simulink model "RL_TTS3_System_Blank"  (R2019b)
settings: Solver=FixedStepAuto  StartTime=0.0  StopTime=10.0  FixedStep=0.01  RelTol=1e-3
undefined symbols (not defined in the file or in its folder): tubeSpeed1, tubeSpeed2
settings Model: Creator=rdkluijv  LastModifiedBy=edtve
settings DebuggingCC: BusObjectLabelMismatch=none
settings SFSimCC: CustomCodeUndefinedFunction=UseInterfaceOnly
settings CodeAppCC: MaxIdLength=63

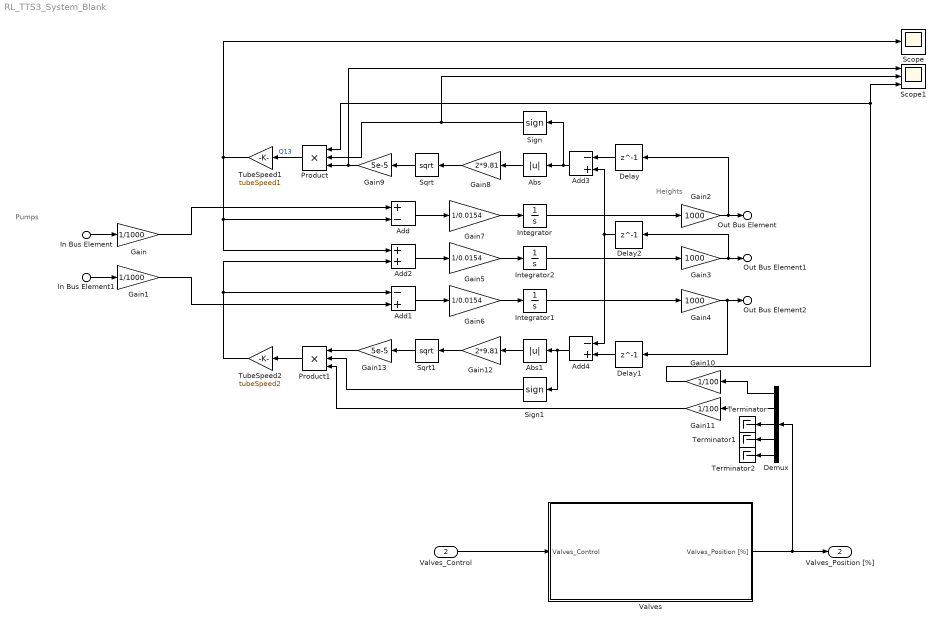
== system RL_TTS3_System_Blank ==
  note: Heights
  note: Pumps
  In Bus Element : Inport  PortName=Pumps [l/s]  Element=Left
  In Bus Element1 : Inport  PortName=Pumps [l/s]  Element=Right
  Valves_Control : Inport  Port=2  OutDataTypeStr=Bus: ValvesSICO
  Abs : Abs
  Abs1 : Abs
  Add : Sum  Inputs=+-
  Add1 : Sum  Inputs=-+
  Add2 : Sum
  Add3 : Sum  Inputs=-+
  Add4 : Sum  Inputs=-+
  Delay : Delay  DelayLength=1
  Delay1 : Delay  DelayLength=1
  Delay2 : Delay  DelayLength=1
  Demux : Demux  Outputs=5
  Gain : Gain  Gain=1/1000
  Gain1 : Gain  Gain=1/1000
  Gain10 : Gain  Gain=1/100
  Gain11 : Gain  Gain=1/100
  Gain12 : Gain  Gain=2*9.81
  Gain13 : Gain  Gain=5e-5
  Gain2 : Gain  Gain=1000
  Gain3 : Gain  Gain=1000
  Gain4 : Gain  Gain=1000
  Gain5 : Gain  Gain=1/0.0154
  Gain6 : Gain  Gain=1/0.0154
  Gain7 : Gain  Gain=1/0.0154
  Gain8 : Gain  Gain=2*9.81
  Gain9 : Gain  Gain=5e-5
  Integrator : Integrator
  Integrator1 : Integrator
  Integrator2 : Integrator
  Product : Product  Inputs=3
  Product1 : Product  Inputs=3
  Scope : Scope
  Scope1 : Scope  NumInputPorts=3
  Sign : Signum
  Sign1 : Signum
  Sqrt : Sqrt  SaturateOnIntegerOverflow=on
  Sqrt1 : Sqrt  SaturateOnIntegerOverflow=on
  Terminator : Terminator
  Terminator1 : Terminator
  Terminator2 : Terminator
  TubeSpeed1 : Gain  Gain=tubeSpeed1
  TubeSpeed2 : Gain  Gain=tubeSpeed2
  Valves : Subsystem  TreatAsAtomicUnit=on
  Out Bus Element : Outport  VectorParamsAs1DForOutWhenUnconnected=off  PortName=Heights [mm]  Element=Left
  Out Bus Element1 : Outport  VectorParamsAs1DForOutWhenUnconnected=off  PortName=Heights [mm]  Element=Middle
  Out Bus Element2 : Outport  VectorParamsAs1DForOutWhenUnconnected=off  PortName=Heights [mm]  Element=Right
  Valves_Position [%] : Outport  Port=2  OutDataTypeStr=Bus: ValvesSOCI
  wires:
  Valves_Control/1 -> Valves/1(Valves_Control)
  Valves/1(Valves_Position [%]) -> Demux/1, Valves_Position [%]/1
  In Bus Element/1 -> Gain/1
  In Bus Element1/1 -> Gain1/1
  Gain4/1 -> Delay1/1, Out Bus Element2/1
  Gain3/1 -> Delay2/1, Out Bus Element1/1
  Gain2/1 -> Delay/1, Out Bus Element/1
  Product1/1 -> TubeSpeed2/1
  Add2/1 -> Gain5/1
  Add1/1 -> Gain6/1
  Add/1 -> Gain7/1
  Gain7/1 -> Integrator/1
  Gain6/1 -> Integrator1/1
  Gain5/1 -> Integrator2/1
  Gain/1 -> Add/1
  Delay/1 -> Add3/1
  Add3/1 -> Sign/1, Abs/1
  Gain8/1 -> Sqrt/1
  Sqrt/1 -> Gain9/1
  Demux/3 -> Terminator/1
  Demux/4 -> Terminator1/1
  Demux/5 -> Terminator2/1
  Demux/1 -> Gain10/1
  Demux/2 -> Gain11/1
  Gain9/1 -> Product/3, Scope1/1
  Gain10/1 -> Scope1/3, Product/1
  Product/1 -> TubeSpeed1/1  "Q13"
  Add4/1 -> Sign1/1, Abs1/1
  Gain12/1 -> Sqrt1/1
  Sqrt1/1 -> Gain13/1
  Gain13/1 -> Product1/1
  Integrator/1 -> Gain2/1
  Abs/1 -> Gain8/1
  Abs1/1 -> Gain12/1
  Sign/1 -> Scope1/2, Product/2
  Sign1/1 -> Product1/2
  Integrator2/1 -> Gain3/1
  Integrator1/1 -> Gain4/1
  Delay2/1 -> Add4/1, Add3/2
  Delay1/1 -> Add4/2
  Gain11/1 -> Product1/3
  Gain1/1 -> Add1/2
  TubeSpeed2/1 -> Add2/2, Add1/1
  TubeSpeed1/1 -> Scope/1, Add/2, Add2/1

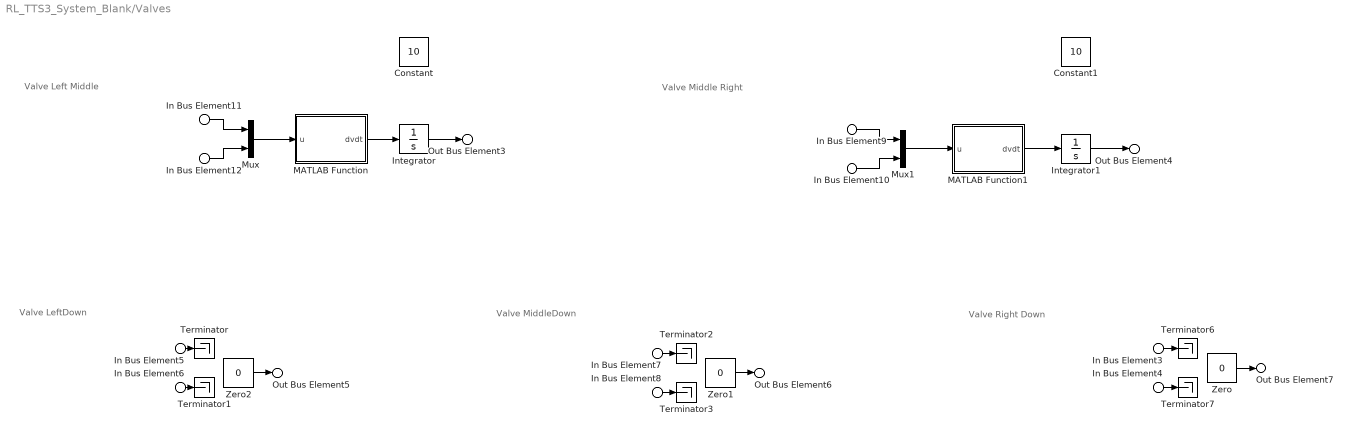
== system RL_TTS3_System_Blank/Valves ==
  note: Valve Right Down
  note: Valve Left Middle
  note: Valve Middle Right
  note: Valve MiddleDown
  note: Valve LeftDown
  In Bus Element3 : Inport  PortName=Valves_Control  Element=RightDown.Open
  In Bus Element4 : Inport  PortName=Valves_Control  Element=RightDown.Close
  In Bus Element5 : Inport  PortName=Valves_Control  Element=LeftDown.Open
  In Bus Element6 : Inport  PortName=Valves_Control  Element=LeftDown.Close
  In Bus Element7 : Inport  PortName=Valves_Control  Element=MiddleDown.Open
  In Bus Element8 : Inport  PortName=Valves_Control  Element=MiddleDown.Close
  In Bus Element9 : Inport  PortName=Valves_Control  Element=MiddleRight.Open
  In Bus Element10 : Inport  PortName=Valves_Control  Element=MiddleRight.Close
  In Bus Element11 : Inport  PortName=Valves_Control  Element=LeftMiddle.Open
  In Bus Element12 : Inport  PortName=Valves_Control  Element=LeftMiddle.Close
  Constant : Constant  Value=10
  Constant1 : Constant  Value=10
  Integrator : Integrator
  Integrator1 : Integrator
  MATLAB Function : MATLAB Function  TreatAsAtomicUnit=on
  MATLAB Function1 : MATLAB Function  TreatAsAtomicUnit=on
  Mux : Mux  Inputs=2
  Mux1 : Mux  Inputs=2
  Terminator{,1..3,6..7} (6 alike) : Terminator
  Zero : Constant  Value=0  OutDataTypeStr=Inherit: Inherit via back propagation
  Zero1 : Constant  Value=0  OutDataTypeStr=Inherit: Inherit via back propagation
  Zero2 : Constant  Value=0  OutDataTypeStr=Inherit: Inherit via back propagation
  Out Bus Element3 : Outport  VectorParamsAs1DForOutWhenUnconnected=off  PortName=Valves_Position [%]  Element=LeftMiddle
  Out Bus Element4 : Outport  VectorParamsAs1DForOutWhenUnconnected=off  PortName=Valves_Position [%]  Element=MiddleRight
  Out Bus Element5 : Outport  VectorParamsAs1DForOutWhenUnconnected=off  PortName=Valves_Position [%]  Element=LeftDown
  Out Bus Element6 : Outport  VectorParamsAs1DForOutWhenUnconnected=off  PortName=Valves_Position [%]  Element=MiddleDown
  Out Bus Element7 : Outport  VectorParamsAs1DForOutWhenUnconnected=off  PortName=Valves_Position [%]  Element=RightDown
  wires:
  Zero/1 -> Out Bus Element7/1
  Zero1/1 -> Out Bus Element6/1
  Zero2/1 -> Out Bus Element5/1
  In Bus Element5/1 -> Terminator/1
  In Bus Element6/1 -> Terminator1/1
  In Bus Element7/1 -> Terminator2/1
  In Bus Element8/1 -> Terminator3/1
  In Bus Element3/1 -> Terminator6/1
  In Bus Element4/1 -> Terminator7/1
  MATLAB Function/1(dvdt) -> Integrator/1
  MATLAB Function1/1(dvdt) -> Integrator1/1
  In Bus Element11/1 -> Mux/1
  Mux/1 -> MATLAB Function/1(u)
  In Bus Element12/1 -> Mux/2
  Mux1/1 -> MATLAB Function1/1(u)
  In Bus Element9/1 -> Mux1/1
  In Bus Element10/1 -> Mux1/2
  Integrator/1 -> Out Bus Element3/1
  Integrator1/1 -> Out Bus Element4/1

== matlab function RL_TTS3_System_Blank/Valves/MATLAB Function1 ==
  data: u input; dvdt output
function dvdt = fcn(u)

    if u(1)==false && u(2)==false
        dvdt = 0;
    elseif u(1)==false && u(2)==true
        dvdt = -100/9;
    elseif u(1)==true && u(2)==false
        dvdt = 100/9;
    else
        dvdt=0;
    end
    
end

== matlab function RL_TTS3_System_Blank/Valves/MATLAB Function ==
  data: u input; dvdt output
function dvdt = fcn(u)

    if u(1)==false && u(2)==false
        dvdt = 0;
    elseif u(1)==false && u(2)==true
        dvdt = -100/9;
    elseif u(1)==true && u(2)==false
        dvdt = 100/9;
    else
        dvdt=0;
    end
    
end
